simulink model "test"  (R2015a)
settings: Solver=ode3  StartTime=0.0  StopTime=50.0  RelTol=1e-3
values from neighbouring files (symbols this model uses):
  A = [3.00381913604 1 0 0 -3.20283559795 0 1 0 1.37849655603 0 0 1 ... (16 elements, 4x4)]    [small_workspace _part1.mat]    (also in whole_data.mat)
  B = [1 0 0 0]    [small_workspace _part1.mat]    (also in whole_data.mat)
  C = [-0.0102732637747 0.0206943191128 0 0]    [small_workspace _part1.mat]    (also in whole_data.mat)
  K = [0.041647581601 -0.0827175020793 0.0491205840961 -0.00732898560866]    [whole_data.mat]
  Ke = 1.51    [Controller_Design.m]    (also in Controller_Design_Real.m; whole_data.mat)
  Kp = 35.3    [Controller_Design.m]    (also in Controller_Design_Real.m; whole_data.mat)
  M = [90.6770554151 70.6684456681 51.7469385594 34.9486926521]    [whole_data.mat]
  Nbar = inv(C*inv(eye(size(A))-A+B*K)*B)    [Controller_Design.m]    (also in Controller_Design_Real.m; whole_data.mat = 0.0692519121834)
undefined symbols (not defined in the file or in its folder): MIO, National_Instruments, PCI
libraries: sldrtlib x3
settings Model: SimulationMode=external  ExtModeTrigDuration=100001  Creator=alunos  LastModifiedBy=alunos
settings DataIOCC: LimitDataPoints=off
settings HardwareCC: ProdIntDivRoundTo=Zero  ProdEndianess=LittleEndian  ProdHWDeviceType=Intel->x86/Pentium  TargetIntDivRoundTo=Zero  TargetEndianess=LittleEndian  TargetHWDeviceType=Intel->x86/Pentium
settings RTWCC: SystemTargetFile=rtwin.tlc  TemplateMakefile=rtwin.tmf  Description=Simulink Desktop Real-Time  RTWCompilerOptimization=on
settings CodeAppCC: MaxIdLength=95
settings RTWinTargetCC: TargetPreCompLibLocation=C:\Program Files\MATLAB\R2015a\toolbox\sldrt\lib\win32

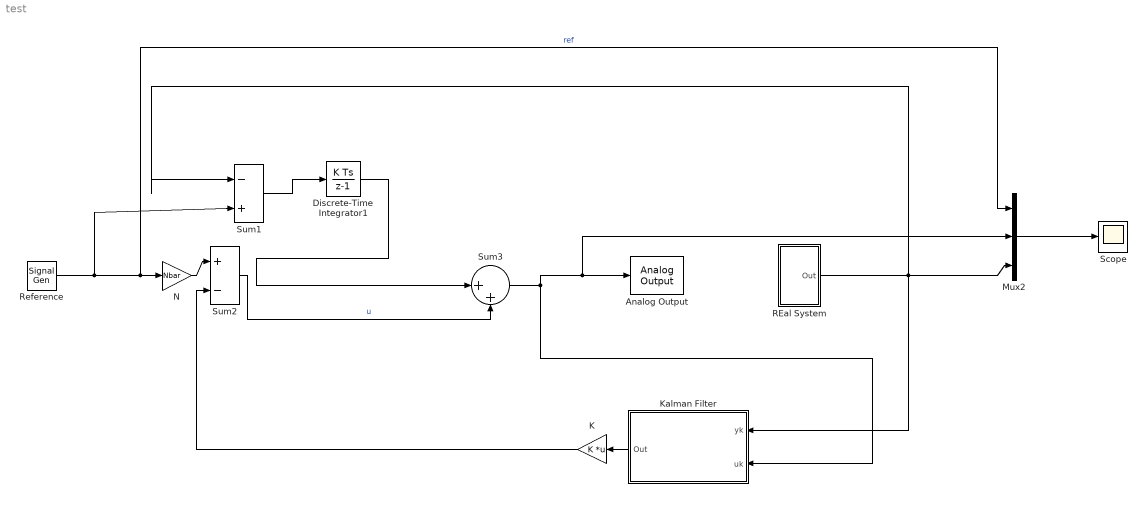
== system test ==
  Analog Output : sldrtlib/Analog Output  SampleTime=0.001  MaxMissedTicks=10  ShowMissedTicks=off  YieldWhenWaiting=off  DrvName=National_Instruments/PCI-MIO-16E-4  DrvAddress=4294967295  DrvOptions=[0 0 0 0 0 0]  Channels=1  RangeMode=1  VoltRange=1  InitialValue=0  FinalValue=0
      settings: AttributesFormatString=National Instruments\nPCI-MIO-16E-4 [auto]
  Discrete-Time Integrator1 : DiscreteIntegrator  gainval=0.05  InitialConditionSetting=State (most efficient)  SampleTime=0.001
  K : Gain  Gain=K  Multiplication=Matrix(K*u)
  Kalman Filter : Subsystem
  Mux2 : Mux  Inputs=3
  N : Gain  Gain=Nbar
  "REal System " : Subsystem
  Reference : SignalGenerator  WaveForm=square  Amplitude=30  Frequency=0.2
  Scope : Scope
      settings: ShowLegends=on  YMin=-35  YMax=35
  Sum1 : Sum  Inputs=|-+
  Sum2 : Sum  Inputs=|+-
  Sum3 : Sum  Inputs=|++
  wires:
  N/1 -> Sum2/1
  Reference/1 -> Sum1/2, Mux2/1, N/1  "ref"
  Mux2/1 -> Scope/1
  Kalman Filter/1(Out) -> K/1
  "REal System "/1(Out) -> Kalman Filter/1("yk "), Sum1/1, Mux2/3
  K/1 -> Sum2/2
  Sum3/1 -> Analog Output/1, Mux2/2, Kalman Filter/2("uk ")
  Sum2/1 -> Sum3/2  "u"
  Sum1/1 -> Discrete-Time Integrator1/1
  Discrete-Time Integrator1/1 -> Sum3/1

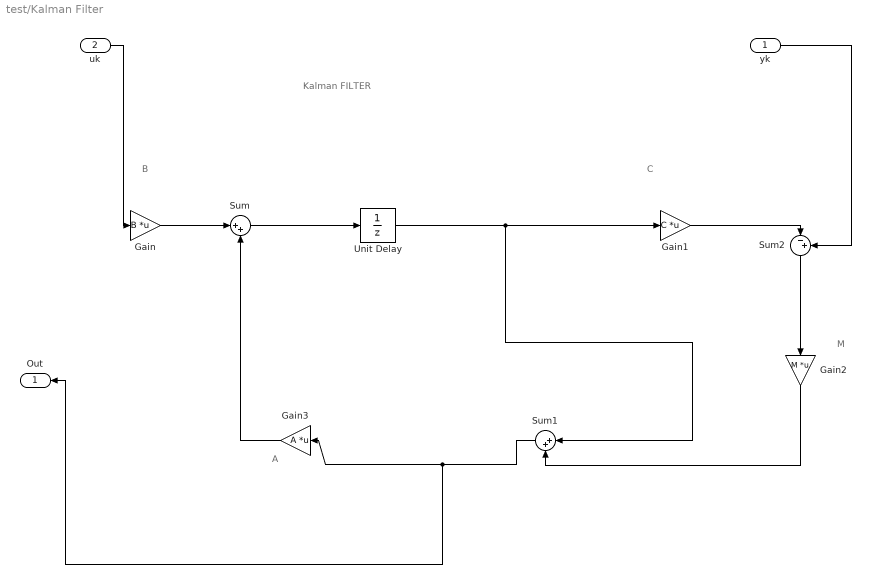
== system test/Kalman Filter ==
  note: A
  note: B
  note: C
  note: M
  note: Kalman FILTER
  "yk " : Inport
  "uk " : Inport  Port=2
  Gain : Gain  Gain=B  Multiplication=Matrix(K*u)
  Gain1 : Gain  Gain=C  Multiplication=Matrix(K*u)
  Gain2 : Gain  Gain=M  Multiplication=Matrix(K*u)
  Gain3 : Gain  Gain=A  Multiplication=Matrix(K*u)
  Sum : Sum  Inputs=|++
  Sum1 : Sum  Inputs=|++
  Sum2 : Sum  Inputs=|-+
  Unit Delay : UnitDelay  SampleTime=-1
  Out : Outport
  wires:
  Sum1/1 -> Gain3/1, Out/1
  Sum2/1 -> Gain2/1
  "uk "/1 -> Gain/1
  Gain3/1 -> Sum/2
  Sum/1 -> Unit Delay/1
  Gain/1 -> Sum/1
  Unit Delay/1 -> Gain1/1, Sum1/1
  "yk "/1 -> Sum2/2
  Gain2/1 -> Sum1/2
  Gain1/1 -> Sum2/1

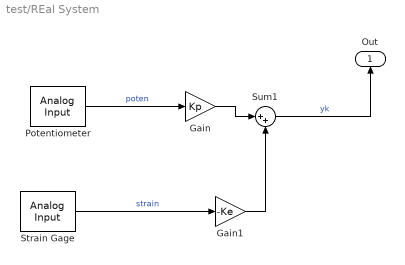
== system test/REal System  ==
  Gain : Gain  Gain=Kp
  Gain1 : Gain  Gain=-Ke
  Potentiometer : sldrtlib/Analog Input  SampleTime=0.001  MaxMissedTicks=10  ShowMissedTicks=off  YieldWhenWaiting=off  DrvName=National_Instruments/PCI-MIO-16E-4  DrvAddress=4294967295  DrvOptions=[0 0 0 0 0 0]  Channels=1  RangeMode=1  VoltRange=1  DataType=1
      settings: AttributesFormatString=National Instruments\nPCI-MIO-16E-4 [auto]
  Strain Gage : sldrtlib/Analog Input  SampleTime=0.001  MaxMissedTicks=10  ShowMissedTicks=off  YieldWhenWaiting=off  DrvName=National_Instruments/PCI-MIO-16E-4  DrvAddress=4294967295  DrvOptions=[0 0 0 0 0 0]  Channels=2  RangeMode=1  VoltRange=1  DataType=1
      settings: AttributesFormatString=National Instruments\nPCI-MIO-16E-4 [auto]
  Sum1 : Sum  Inputs=|++
  Out : Outport
  wires:
  Potentiometer/1 -> Gain/1  "poten"
  Strain Gage/1 -> Gain1/1  "strain"
  Sum1/1 -> Out/1  "yk"
  Gain/1 -> Sum1/1
  Gain1/1 -> Sum1/2
